simulink model "planta"  (R2015a)
settings: Solver=ode1  StartTime=0.0  StopTime=Tsimu  FixedStep=p  RelTol=1e-3
values from neighbouring files (symbols this model uses):
  A = [(rgo*Cwro2 - Cwpg2) (rgo*Cwro3 - Cwpg3); (Cwro2 - Cwpo2) (Cwro3 - Cwpo3)]    [init.m]
  a0 = r0    (= 4252610.83744)    [init.m]
  B = [1 0]'    [init.m]
  C = g/Aw*[1 1]    [init.m]
  f0 = 62.8/20*2    (= 6.28)    [init.m]
  G = eye(2)    [init.m]
  h = 50    [init.m]
  K0 = place(A, B, [-0.5 -0.001])    [init.m]
  L = (place(A',C',Lp))'    [init.m]
  N0 = 1/(C*inv(-1*(A - B*K0))*B)    [init.m]
  P0 = eye(2)*10e3    [init.m]
  Qn = eye(2)*10e10    [init.m]
  R = 10    [init.m]
  r0 = g/Aw*(12e3 + 76e3)    (= 4252610.83744)    [init.m]
  Tsimu = 10e3    (= 10000)    [init.m]
  x0 = [5e4 5e4]'*1    [init.m]
  x0hat = x0    [init.m]
  xHatInit = x0 + (randn(2)*[1 0]')*10e3    [init.m]
undefined symbols (not defined in the file or in its folder): Cd, H, phi
libraries: dspinverses x2, simulink x1, dspsrcs4 x1
settings Model: Creator=alessandropeixoto  LastModifiedBy=Raposo
settings SolverCC: AutoInsertRateTranBlk=on
settings DataIOCC: SaveFormat=Dataset
settings HardwareCC: ProdBitPerPointer=64  ProdLargestAtomicFloat=Float  ProdIntDivRoundTo=Zero  ProdEndianess=LittleEndian  ProdHWDeviceType=Specified
settings GRTTargetCC: GeneratePreprocessorConditionals=Use local settings

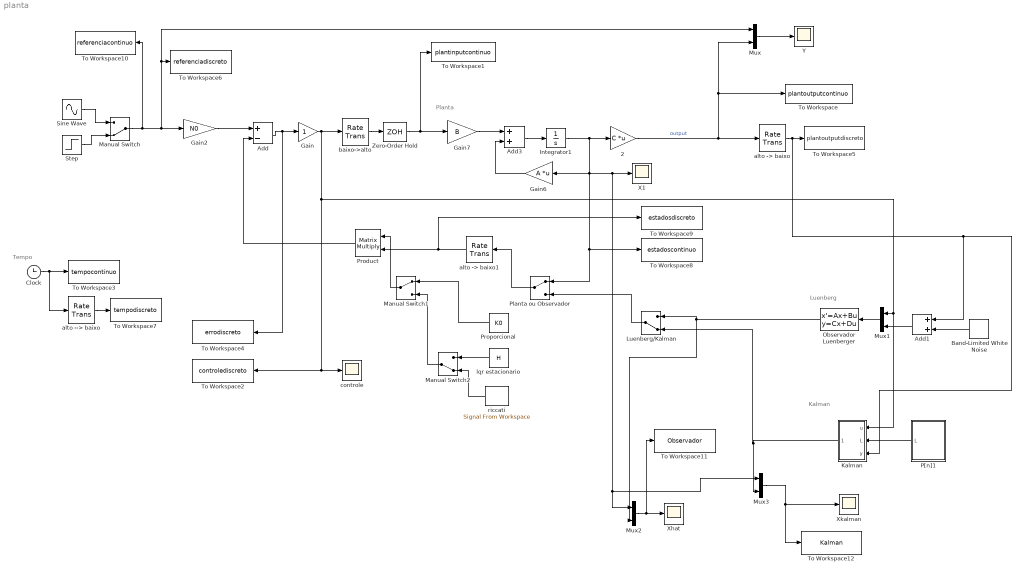
== system planta ==
  note: Kalman
  note: Luenberg
  note: Tempo
  note: Planta
  " 2" : Gain  Gain=C  Multiplication=Matrix(K*u)
  Add : Sum  Inputs=+-
  Add1 : Sum
  Add3 : Sum
  Band-Limited White Noise : simulink/Sources/Band-Limited White Noise  Cov=vk  Ts=h  seed=[23341]
  Clock : Clock
  Gain : Gain
  Gain2 : Gain  Gain=N0
  Gain6 : Gain  Gain=A  Multiplication=Matrix(K*u)
  Gain7 : Gain  Gain=B
  Integrator1 : Integrator  InitialCondition=x0
  "Kalman " : Subsystem
  Luenberg/Kalman : ManualSwitch  CurrentSetting=0
  Manual Switch : ManualSwitch  CurrentSetting=0
  Manual Switch1 : ManualSwitch
  Manual Switch2 : ManualSwitch  CurrentSetting=0
  Mux{,1..3} (4 alike) : Mux  Inputs=2
  Observador Luenberger : StateSpace  A=A - L*C  B=[B L]  C=eye(2,2)  D=zeros(2,2)  X0=xHatInit
  P[n]1 : Subsystem
  Planta ou Observador : ManualSwitch
  Product : Product  Multiplication=Matrix(*)
  Proporcional : Constant  Value=K0  SampleTime=h
  Sine Wave : Sin  Amplitude=a0  Frequency=f0  SampleTime=h
  Step : Step  Time=Tsimu/2  After=r0  SampleTime=h
  To Workspace : ToWorkspace  VariableName=plantoutputcontinuo  SampleTime=-1
      settings: Save2DSignal=2-D array (concatenate along first dimension)
  To Workspace1 : ToWorkspace  VariableName=plantinputcontinuo  SampleTime=-1
  To Workspace10 : ToWorkspace  VariableName=referenciacontinuo  SampleTime=1
      settings: Save2DSignal=2-D array (concatenate along first dimension)
  To Workspace11 : ToWorkspace  VariableName=Observador  SaveFormat=Timeseries  SampleTime=1
  To Workspace12 : ToWorkspace  VariableName=Kalman  SaveFormat=Timeseries  SampleTime=1
  To Workspace2 : ToWorkspace  VariableName=controlediscreto  SampleTime=h
  To Workspace3 : ToWorkspace  VariableName=tempocontinuo  SampleTime=-1
  To Workspace4 : ToWorkspace  VariableName=errodiscreto  SampleTime=h
  To Workspace5 : ToWorkspace  VariableName=plantoutputdiscreto  SampleTime=h
      settings: Save2DSignal=2-D array (concatenate along first dimension)
  To Workspace6 : ToWorkspace  VariableName=referenciadiscreto  SampleTime=h
      settings: Save2DSignal=2-D array (concatenate along first dimension)
  To Workspace7 : ToWorkspace  VariableName=tempodiscreto  SampleTime=h
  To Workspace8 : ToWorkspace  VariableName=estadoscontinuo  SampleTime=1
  To Workspace9 : ToWorkspace  VariableName=estadosdiscreto  SampleTime=h
  X1 : Scope
      settings: TimeRange=auto  ShowLegends=on  MaxDataPoints=5000  SaveToWorkspace=off  SaveName=ScopeData3  YMin=-46723.51338  YMax=141310.45653  SampleTime=-1
  Xhat : Scope
      settings: TimeRange=auto  ShowLegends=on  MaxDataPoints=5000  SaveToWorkspace=off  SaveName=ScopeData2  YMin=-56673.96328  YMax=120355.12119  SampleTime=-1
  Xkalman : Scope
      settings: TimeRange=auto  ShowLegends=on  MaxDataPoints=5000  SaveToWorkspace=off  YMin=-336415.79953  YMax=157247.31941  SampleTime=-1
  Y : Scope
      settings: TimeRange=auto  ShowLegends=on  MaxDataPoints=5000  SaveToWorkspace=off  SaveName=ScopeData  YMin=-1842447.33144  YMax=5574174.49824  SampleTime=-1
  Zero-Order Hold : ZeroOrderHold  SampleTime=-1
  alto --> baixo : RateTransition  OutPortSampleTime=h
  "alto -> baixo" : RateTransition  OutPortSampleTime=h
  "alto -> baixo1" : RateTransition  OutPortSampleTime=h
  baixo->alto : RateTransition  OutPortSampleTime=h
  controle : Scope
      settings: TimeRange=auto  ShowLegends=on  MaxDataPoints=5000  SaveToWorkspace=off  YMin=-53.58697  YMax=5.95411  SampleTime=-1
  lqr estacionario : Constant  Value=H  SampleTime=h
  riccati : dspsrcs4/Signal From Workspace  X=lx'  Ts=h  nsamps=1  OutputAfterFinalValue=Setting to zero  ignoreOrWarnInputAndFrameLengths=off
  wires:
  Gain/1 -> "Kalman "/1(u), Mux1/1, controle/1, To Workspace2/1, baixo->alto/1
  Add/1 -> Gain/1, To Workspace4/1
  Clock/1 -> alto --> baixo/1, To Workspace3/1
  alto --> baixo/1 -> To Workspace7/1
  baixo->alto/1 -> Zero-Order Hold/1
  "alto -> baixo"/1 -> "Kalman "/3("y "), Add1/1, To Workspace5/1
  Sine Wave/1 -> Manual Switch/1
  Step/1 -> Manual Switch/2
  Manual Switch/1 -> To Workspace10/1, Mux/1, To Workspace6/1, Gain2/1
  Gain7/1 -> Add3/1
  Add3/1 -> Integrator1/1
  Zero-Order Hold/1 -> To Workspace1/1, Gain7/1
  Integrator1/1 -> To Workspace8/1, Planta ou Observador/1, Mux3/1, Mux2/1, X1/1, Gain6/1, " 2"/1
  " 2"/1 -> Mux/2, To Workspace/1, "alto -> baixo"/1  "output"
  Gain6/1 -> Add3/2
  "alto -> baixo1"/1 -> Product/2, To Workspace9/1
  Mux/1 -> Y/1
  Product/1 -> Add/2
  Proporcional/1 -> Manual Switch1/1
  Manual Switch2/1 -> Manual Switch1/2
  lqr estacionario/1 -> Manual Switch2/1
  riccati/1 -> Manual Switch2/2
  Manual Switch1/1 -> Product/1
  Mux1/1 -> Observador Luenberger/1
  Planta ou Observador/1 -> "alto -> baixo1"/1
  Mux2/1 -> To Workspace11/1, Xhat/1
  Add1/1 -> Mux1/2
  Band-Limited White Noise/1 -> Add1/2
  P[n]1/1(L) -> "Kalman "/2(L)
  Luenberg/Kalman/1 -> Planta ou Observador/2
  Observador Luenberger/1 -> Mux2/2, Luenberg/Kalman/1
  Gain2/1 -> Add/1
  Mux3/1 -> To Workspace12/1, Xkalman/1
  "Kalman "/1(Out1) -> Mux3/2, Luenberg/Kalman/2

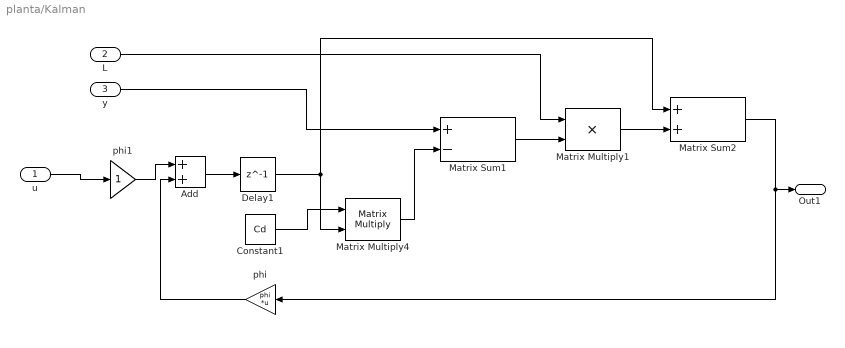
== system planta/Kalman  ==
  u : Inport
  L : Inport  Port=2
  "y " : Inport  Port=3
  Add : Sum
  Constant1 : Constant  Value=Cd  VectorParams1D=off  SampleTime=-1
  Delay1 : Delay  DelayLength=1  InitialCondition=x0hat
  Matrix Sum1 : Sum  Inputs=+-
  Matrix Sum2 : Sum
  Matrix Multiply1 : Product  Inputs=**
  Matrix Multiply4 : Product  Inputs=**  Multiplication=Matrix(*)
  phi : Gain  Gain=phi  Multiplication=Matrix(K*u)
  phi1 : Gain
  Out1 : Outport
  wires:
  phi/1 -> Add/2
  u/1 -> phi1/1
  Add/1 -> Delay1/1
  Matrix Sum2/1 -> Out1/1, phi/1
  "y "/1 -> Matrix Sum1/1
  Delay1/1 -> Matrix Multiply4/2, Matrix Sum2/1
  L/1 -> Matrix Multiply1/1
  Constant1/1 -> Matrix Multiply4/1
  Matrix Multiply4/1 -> Matrix Sum1/2
  Matrix Sum1/1 -> Matrix Multiply1/2
  Matrix Multiply1/1 -> Matrix Sum2/2
  phi1/1 -> Add/1

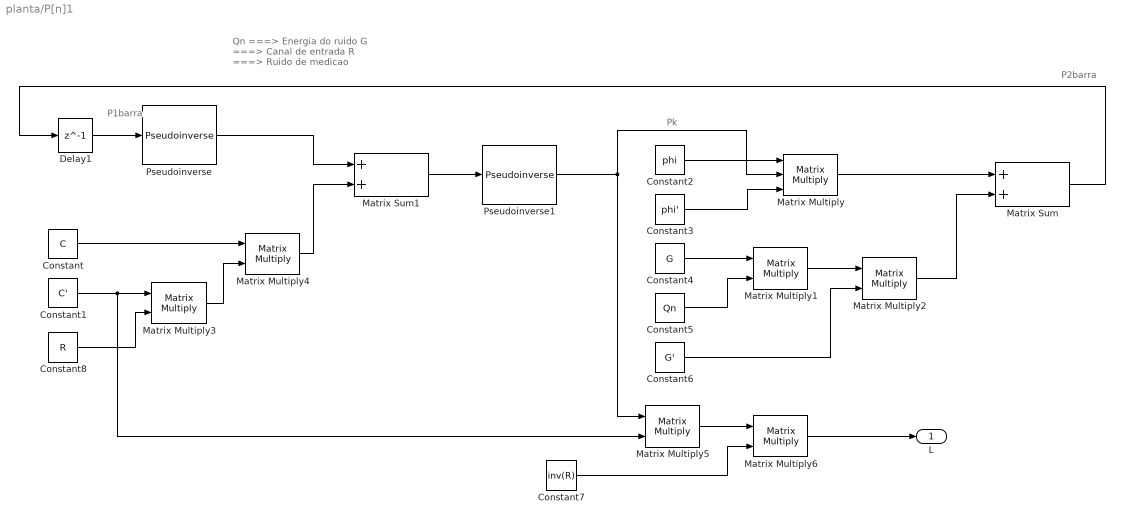
== system planta/P[n]1 ==
  note: Pk
  note: Qn ===> Energia do ruido
      | G   ===> Canal de entrada
      | R   ===> Ruido de medicao
  note: P2barra
  note: P1barra
  Constant : Constant  Value=C  VectorParams1D=off
  Constant1 : Constant  Value=C'  VectorParams1D=off
  Constant2 : Constant  Value=phi  VectorParams1D=off
  Constant3 : Constant  Value=phi'  VectorParams1D=off
  Constant4 : Constant  Value=G  VectorParams1D=off
  Constant5 : Constant  Value=Qn  VectorParams1D=off
  Constant6 : Constant  Value=G'  VectorParams1D=off
  Constant7 : Constant  Value=inv(R)  VectorParams1D=off
  Constant8 : Constant  Value=R  VectorParams1D=off
  Delay1 : Delay  DelayLength=1  InitialCondition=P0
  Matrix Sum : Sum
  Matrix Sum1 : Sum
  Matrix Multiply : Product  Inputs=***  Multiplication=Matrix(*)
  Matrix Multiply{1..6} (6 alike) : Product  Inputs=**  Multiplication=Matrix(*)
  Pseudoinverse : dspinverses/Pseudoinverse  wanterr=off
  Pseudoinverse1 : dspinverses/Pseudoinverse  wanterr=off
  L : Outport
  wires:
  Pseudoinverse1/1 -> Matrix Multiply5/1, Matrix Multiply/2
  Matrix Sum/1 -> Delay1/1
  Matrix Multiply6/1 -> L/1
  Delay1/1 -> Pseudoinverse/1
  Constant/1 -> Matrix Multiply4/1
  Constant1/1 -> Matrix Multiply5/2, Matrix Multiply3/1
  Constant2/1 -> Matrix Multiply/1
  Constant3/1 -> Matrix Multiply/3
  Constant4/1 -> Matrix Multiply1/1
  Constant5/1 -> Matrix Multiply1/2
  Constant6/1 -> Matrix Multiply2/2
  Matrix Multiply/1 -> Matrix Sum/1
  Matrix Multiply1/1 -> Matrix Multiply2/1
  Matrix Multiply2/1 -> Matrix Sum/2
  Constant8/1 -> Matrix Multiply3/2
  Matrix Multiply3/1 -> Matrix Multiply4/2
  Matrix Multiply4/1 -> Matrix Sum1/2
  Pseudoinverse/1 -> Matrix Sum1/1
  Matrix Sum1/1 -> Pseudoinverse1/1
  Matrix Multiply5/1 -> Matrix Multiply6/1
  Constant7/1 -> Matrix Multiply6/2
